simulink model "s_hover_lqr"  (Simulink 7.7)
settings: Solver=ode4  StartTime=0.0  StopTime=20  FixedStep=0.001  RelTol=1e-3
undefined symbols (not defined in the file or in its folder): CMD_RATE_LIMIT, K, K_AMP, KMIO, V_bias, VMAX_AMP, VMAX_DAC
libraries: simulink_extras x7
settings Model: Creator=hpineros  LastModifiedBy=alumno4  ExtModeTrigDuration=10000  TunableVars=A,B,C,CMD_RATE_LIMIT,D,INT_JOYSTICK_SAT_LOWER,INT_JOYSTICK_SAT_UPPER,JOYSTICK_X_DZ,JOYSTICK_Y_DZ,Jp,Jr,Jy,K,K_AMP,K_EC_P,K_EC_R,K_EC_Y,K_JOYSTICK_X,K_JOYSTICK_Y,Kf,Ktc,Ktn,Q,R,VMAX_AMP,VMAX_DAC,V_bias,g,l,wcf,zetaf  TunableVarsStorageClass=Auto,Auto,Auto,Auto,Auto,Auto,Auto,Auto,Auto,Auto,Auto,Auto,Auto,Auto,Auto,Auto,Auto,Auto,Auto,Auto,Auto,Auto,Auto,Auto,Auto,Auto,Auto,Auto,Auto,Auto,Auto  TunableVarsTypeQualifier=,,,,,,,,,,,,,,,,,,,,,,,,,,,,,,
settings SolverCC: PositivePriorityOrder=on
settings OptimizationCC: InlineParams=on  InitFltsAndDblsToZero=on
settings DebuggingCC: SaveWithParameterizedLinksMsg=none  StrictBusMsg=Warning
settings RTWCC: SystemTargetFile=quarc_windows.tlc  TemplateMakefile=quarc_default_tmf  Description=QuaRC Win32 Target  ProcessScript=quarc_windows_make_rtw_hook
settings STFCustomTargetCC: TargetFcnLib=ansi_tfl_tmw.mat  TargetPreCompLibLocation=C:\PROGRA~2\QUARC\lib\2011a\windows\release  FunctionExecutionProfile=off  GeneratePreprocessorConditionals=Disable all  SystemTargetFile=quarc_windows.tlc
settings GRTTargetCC: TargetFcnLib=ansi_tfl_tmw.mat  TargetPreCompLibLocation=C:\PROGRA~2\QUARC\lib\2011a\windows\release  ParMdlRefBuildCompliant=off  CompOptLevelCompliant=off  MatFileLogging=off  ExtMode=on  ExtModeMexFile=quarc_comm

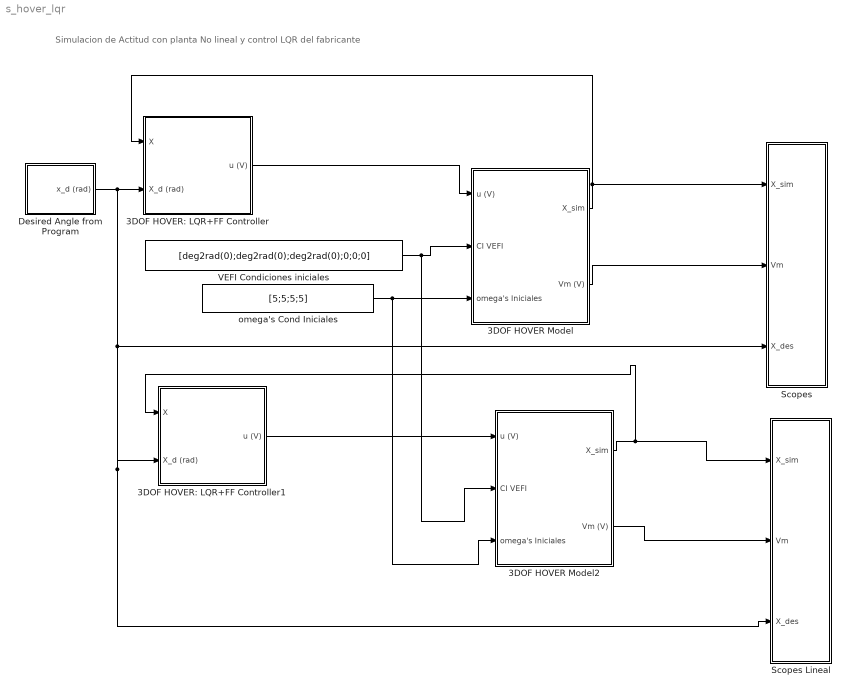
== system s_hover_lqr ==
  note: Simulacion de Actitud con planta No lineal y control LQR del fabricante
  3DOF HOVER Model : Subsystem
  3DOF HOVER Model2 : Subsystem
  3DOF HOVER: LQR+FF Controller : Subsystem
  3DOF HOVER: LQR+FF Controller1 : Subsystem
  Desired Angle from Program : Subsystem
  Scopes : Subsystem
  Scopes Lineal : Subsystem
  VEFI Condiciones iniciales : Constant  Value=[deg2rad(0);deg2rad(0);deg2rad(0);0;0;0]
  omega's Cond Iniciales : Constant  Value=[5;5;5;5]
  wires:
  Desired Angle from Program/1(x_d (rad)) -> 3DOF HOVER: LQR+FF Controller/2(X_d (rad)), Scopes/3(X_des), 3DOF HOVER: LQR+FF Controller1/2(X_d (rad)), Scopes Lineal/3(X_des)
  3DOF HOVER Model/2(Vm (V)) -> Scopes/2(Vm)
  3DOF HOVER: LQR+FF Controller/1(u (V)) -> 3DOF HOVER Model/1(u (V))
  3DOF HOVER Model/1(X_sim) -> Scopes/1(X_sim), 3DOF HOVER: LQR+FF Controller/1(X)
  VEFI Condiciones iniciales/1 -> 3DOF HOVER Model/2(CI VEFI), 3DOF HOVER Model2/2(CI VEFI)
  omega's Cond Iniciales/1 -> 3DOF HOVER Model/3(omega's Iniciales), 3DOF HOVER Model2/3(omega's Iniciales)
  3DOF HOVER Model2/1(X_sim) -> Scopes Lineal/1(X_sim), 3DOF HOVER: LQR+FF Controller1/1(X)
  3DOF HOVER Model2/2(Vm (V)) -> Scopes Lineal/2(Vm)
  3DOF HOVER: LQR+FF Controller1/1(u (V)) -> 3DOF HOVER Model2/1(u (V))

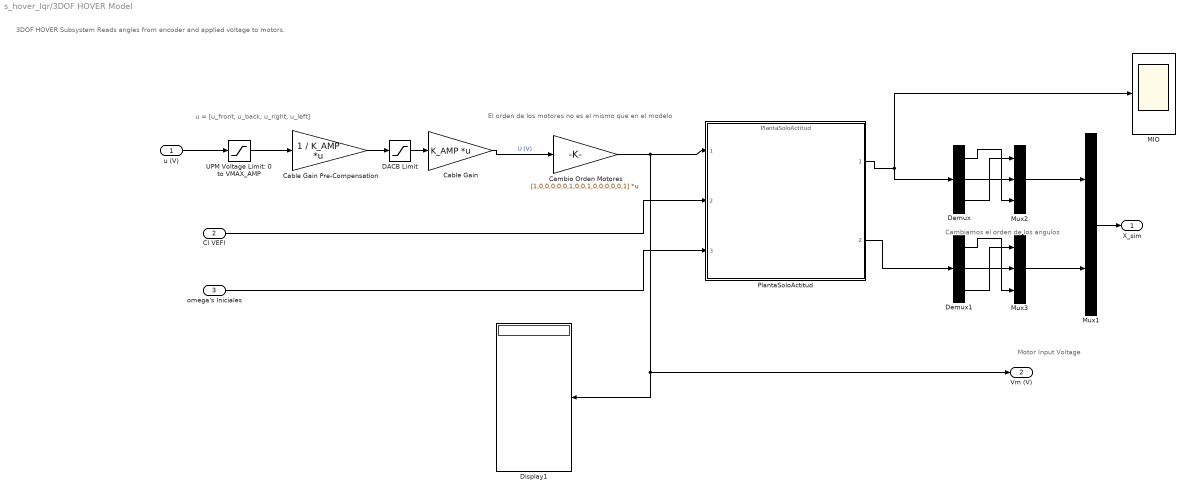
== system s_hover_lqr/3DOF HOVER Model ==
  note: Cambiamos el orden de los angulos
  note: 3DOF HOVER Subsystem
      | Reads angles from encoder and applied voltage to motors.
  note: Motor Input Voltage
  note: u = [u_front, u_back, u_right, u_left]
  note: El orden de los motores no es el mismo que en el modelo
  u (V) : Inport
  CI VEFI : Inport  Port=2
  omega's Iniciales : Inport  Port=3
  Cable Gain : Gain  Gain=K_AMP  Multiplication=Matrix(K*u)  SaturateOnIntegerOverflow=on  OutDataTypeStr=Inherit: Same as input  ParamDataTypeStr=Inherit: Same as input
  Cable Gain Pre-Compensation : Gain  Gain=1 / K_AMP  Multiplication=Matrix(K*u)  SaturateOnIntegerOverflow=on  OutDataTypeStr=Inherit: Same as input  ParamDataTypeStr=Inherit: Same as input
  Cambio Orden Motores : Gain  Gain=[1,0,0,0;0,0,1,0;0,1,0,0;0,0,0,1]  Multiplication=Matrix(K*u)  SaturateOnIntegerOverflow=on  OutDataTypeStr=Inherit: Same as input  ParamDataTypeStr=Inherit: Same as input
  DACB Limit : Saturate  UpperLimit=VMAX_DAC  LowerLimit=-VMAX_DAC
  Demux : Demux  Outputs=3
  Demux1 : Demux  Outputs=3
  Display1 : Display
  "MIO " : Scope
      settings: TickLabels=on  TimeRange=20  YMin=0.00325  YMax=0.0075  DataFormat=Array
  Mux1 : Mux  Inputs=2
  Mux2 : Mux  Inputs=3
  Mux3 : Mux  Inputs=3
  PlantaSoloActitud : ModelReference  ModelNameDialog=PlantaSoloActitud  SimulationMode=Normal  ModelReferenceVersion=1.26  CopyOfModelName=PlantaSoloActitud  DefaultDataLogging=on
  UPM Voltage Limit: 0 to VMAX_AMP : Saturate  UpperLimit=VMAX_AMP  LowerLimit=0
  X_sim : Outport
  Vm (V) : Outport  Port=2
  wires:
  Mux1/1 -> X_sim/1
  Cable Gain/1 -> Cambio Orden Motores/1  "U (V)"
  DACB Limit/1 -> Cable Gain/1
  u (V)/1 -> UPM Voltage Limit: 0 to VMAX_AMP/1
  UPM Voltage Limit: 0 to VMAX_AMP/1 -> Cable Gain Pre-Compensation/1
  Cable Gain Pre-Compensation/1 -> DACB Limit/1
  CI VEFI/1 -> PlantaSoloActitud/2
  omega's Iniciales/1 -> PlantaSoloActitud/3
  PlantaSoloActitud/1 -> "MIO "/1, Demux/1
  PlantaSoloActitud/2 -> Demux1/1
  Demux/2 -> Mux2/2
  Demux/3 -> Mux2/1
  Demux/1 -> Mux2/3
  Demux1/2 -> Mux3/2
  Demux1/3 -> Mux3/1
  Demux1/1 -> Mux3/3
  Mux3/1 -> Mux1/2
  Mux2/1 -> Mux1/1
  Cambio Orden Motores/1 -> PlantaSoloActitud/1, Vm (V)/1, Display1/1

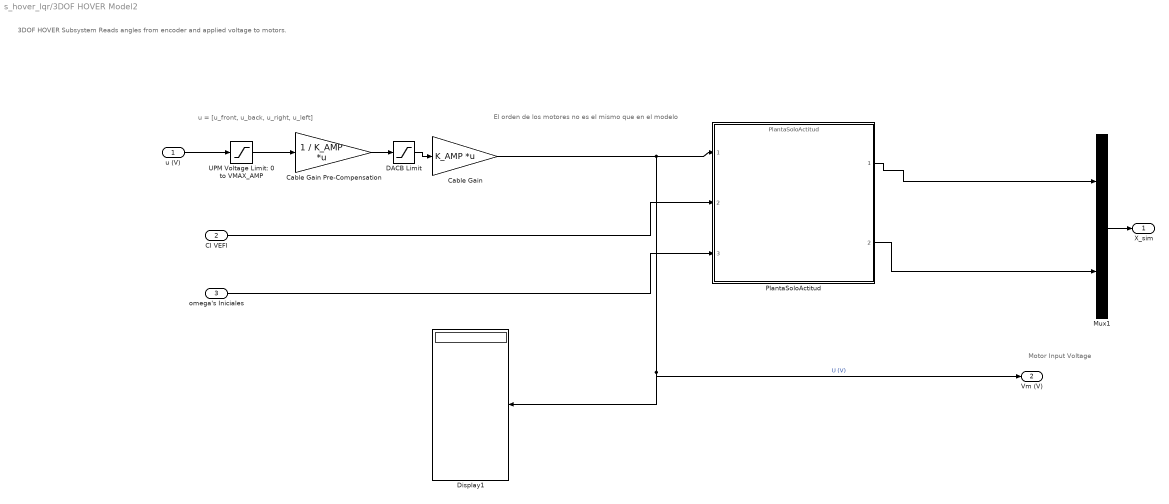
== system s_hover_lqr/3DOF HOVER Model2 ==
  note: 3DOF HOVER Subsystem
      | Reads angles from encoder and applied voltage to motors.
  note: Motor Input Voltage
  note: u = [u_front, u_back, u_right, u_left]
  note: El orden de los motores no es el mismo que en el modelo
  u (V) : Inport
  CI VEFI : Inport  Port=2
  omega's Iniciales : Inport  Port=3
  Cable Gain : Gain  Gain=K_AMP  Multiplication=Matrix(K*u)  SaturateOnIntegerOverflow=on  OutDataTypeStr=Inherit: Same as input  ParamDataTypeStr=Inherit: Same as input
  Cable Gain Pre-Compensation : Gain  Gain=1 / K_AMP  Multiplication=Matrix(K*u)  SaturateOnIntegerOverflow=on  OutDataTypeStr=Inherit: Same as input  ParamDataTypeStr=Inherit: Same as input
  DACB Limit : Saturate  UpperLimit=VMAX_DAC  LowerLimit=-VMAX_DAC
  Display1 : Display
  Mux1 : Mux  Inputs=2
  PlantaSoloActitud : ModelReference  ModelNameDialog=PlantaSoloActitud  SimulationMode=Normal  ModelReferenceVersion=1.26  CopyOfModelName=PlantaSoloActitud  DefaultDataLogging=off
  UPM Voltage Limit: 0 to VMAX_AMP : Saturate  UpperLimit=VMAX_AMP  LowerLimit=0
  X_sim : Outport
  Vm (V) : Outport  Port=2
  wires:
  Mux1/1 -> X_sim/1
  Cable Gain/1 -> PlantaSoloActitud/1, Vm (V)/1, Display1/1  "U (V)"
  DACB Limit/1 -> Cable Gain/1
  u (V)/1 -> UPM Voltage Limit: 0 to VMAX_AMP/1
  UPM Voltage Limit: 0 to VMAX_AMP/1 -> Cable Gain Pre-Compensation/1
  Cable Gain Pre-Compensation/1 -> DACB Limit/1
  CI VEFI/1 -> PlantaSoloActitud/2
  omega's Iniciales/1 -> PlantaSoloActitud/3
  PlantaSoloActitud/1 -> Mux1/1
  PlantaSoloActitud/2 -> Mux1/2

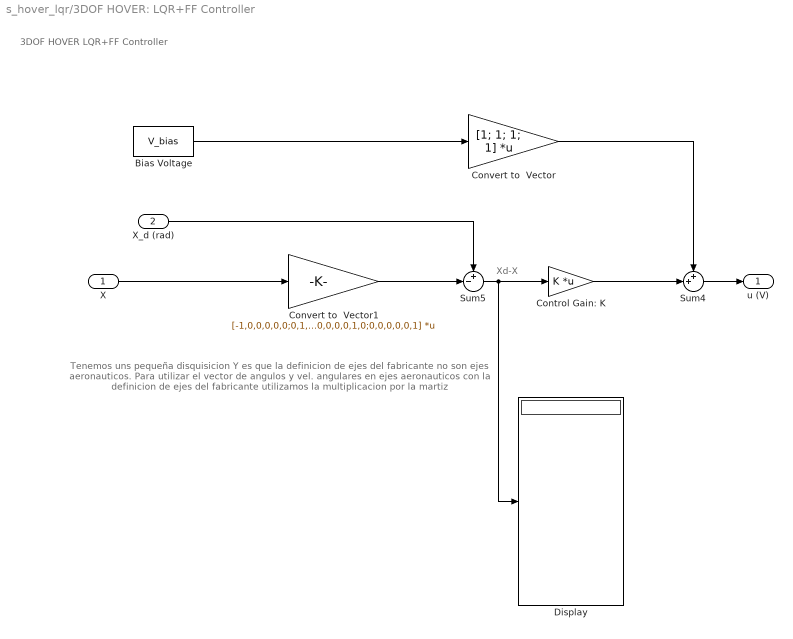
== system s_hover_lqr/3DOF HOVER: LQR+FF Controller ==
  note: Xd-X
  note: 3DOF HOVER LQR+FF Controller
  note: Tenemos uns pequeña disquisicion
      | Y es que la definicion de ejes del fabricante no son ejes aeronauticos.
      | Para utilizar el vector de angulos y vel. angulares en ejes aeronauticos
      | con la definicion de ejes del fabricante utilizamos la multiplicacion por la martiz
  X : Inport
  X_d (rad) : Inport  Port=2
  Bias Voltage : Constant  Value=V_bias
  Control Gain: K : Gain  Gain=K  Multiplication=Matrix(K*u)
  Convert to  Vector : Gain  Gain=[1; 1; 1; 1]  Multiplication=Matrix(K*u)
  Convert to  Vector1 : Gain  Gain=[-1,0,0,0,0,0;0,1,0,0,0,0;0,0,1,0,0,0;0,0,0,-1,0,0;0,0,0,0,1,0;0,0,0,0,0,1]  Multiplication=Matrix(K*u)
  Display : Display
  Sum4 : Sum  Inputs=++|
  Sum5 : Sum  Inputs=+-|
  u (V) : Outport
  wires:
  Sum5/1 -> Control Gain: K/1, Display/1
  X_d (rad)/1 -> Sum5/1
  Convert to  Vector/1 -> Sum4/1
  Control Gain: K/1 -> Sum4/2
  Bias Voltage/1 -> Convert to  Vector/1
  Sum4/1 -> u (V)/1
  Convert to  Vector1/1 -> Sum5/2
  X/1 -> Convert to  Vector1/1

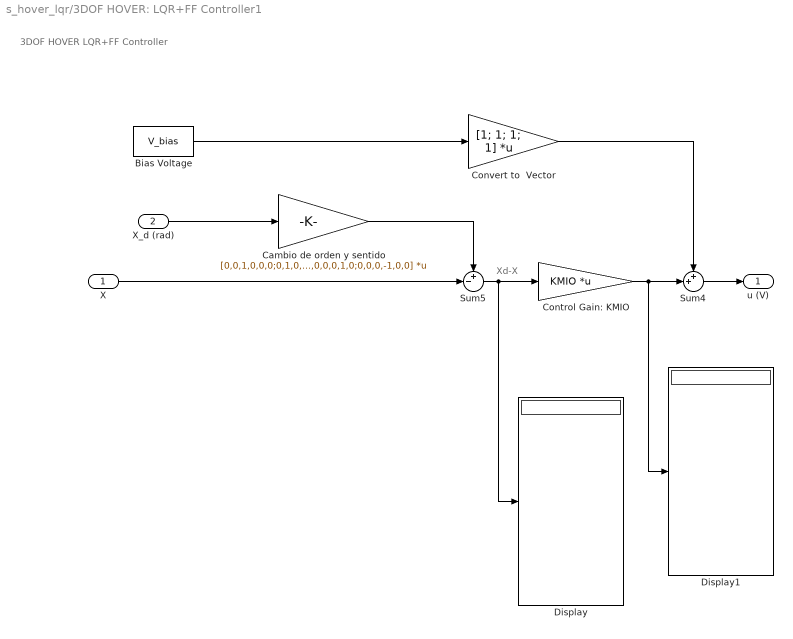
== system s_hover_lqr/3DOF HOVER: LQR+FF Controller1 ==
  note: Xd-X
  note: 3DOF HOVER LQR+FF Controller
  X : Inport
  X_d (rad) : Inport  Port=2
  Bias Voltage : Constant  Value=V_bias
  Cambio de orden y sentido : Gain  Gain=[0,0,1,0,0,0;0,1,0,0,0,0;-1,0,0,0,0,0;0,0,0,0,0,1;0,0,0,0,1,0;0,0,0,-1,0,0]  Multiplication=Matrix(K*u)
  Control Gain: KMIO : Gain  Gain=KMIO  Multiplication=Matrix(K*u) (u vector)
  Convert to  Vector : Gain  Gain=[1; 1; 1; 1]  Multiplication=Matrix(K*u)
  Display : Display
  Display1 : Display
  Sum4 : Sum  Inputs=++|
  Sum5 : Sum  Inputs=+-|
  u (V) : Outport
  wires:
  Sum5/1 -> Control Gain: KMIO/1, Display/1
  X_d (rad)/1 -> Cambio de orden y sentido/1
  Convert to  Vector/1 -> Sum4/1
  Control Gain: KMIO/1 -> Sum4/2, Display1/1
  Bias Voltage/1 -> Convert to  Vector/1
  Sum4/1 -> u (V)/1
  X/1 -> Sum5/2
  Cambio de orden y sentido/1 -> Sum5/1

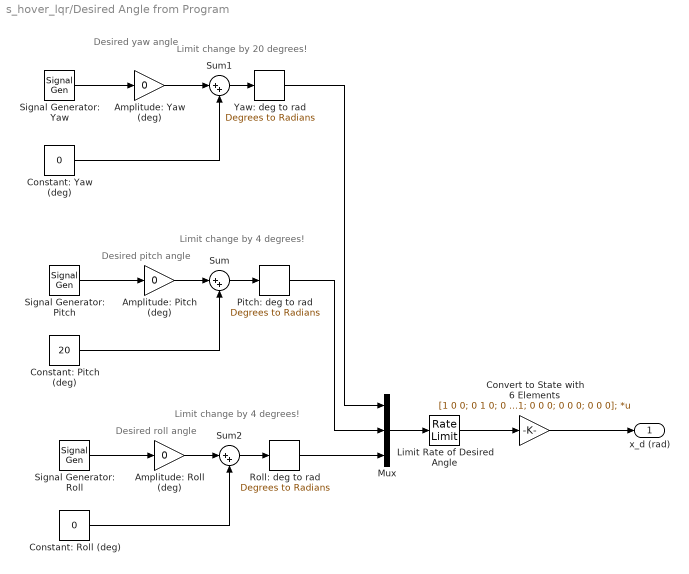
== system s_hover_lqr/Desired Angle from Program ==
  note: Limit change by
      | 4 degrees!
  note: Limit change by
      | 20 degrees!
  note: Limit change by
      | 4 degrees!
  note: Desired roll angle
  note: Desired pitch angle
  note: Desired yaw angle
  Amplitude: Pitch (deg) : Gain  Gain=0
  Amplitude: Roll (deg) : Gain  Gain=0
  Amplitude: Yaw (deg) : Gain  Gain=0
  Constant: Pitch (deg) : Constant  Value=20
  Constant: Roll (deg) : Constant  Value=0
  Constant: Yaw (deg) : Constant  Value=0
  Convert to State with 6 Elements : Gain  Gain=[1 0 0; 0 1 0; 0 0 1; 0 0 0; 0 0 0; 0 0 0];  Multiplication=Matrix(K*u)
  Limit Rate of Desired Angle : RateLimiter  RisingSlewLimit=CMD_RATE_LIMIT  FallingSlewLimit=-CMD_RATE_LIMIT
  Mux : Mux  Inputs=3
  Pitch: deg to rad : simulink_extras/Transformations/Degrees to Radians  SystemSampleTime=-1
  Roll: deg to rad : simulink_extras/Transformations/Degrees to Radians  SystemSampleTime=-1
  Signal Generator: Pitch : SignalGenerator  WaveForm=square  Frequency=0.0000001
  Signal Generator: Roll : SignalGenerator  WaveForm=square  Frequency=0.08
  Signal Generator: Yaw : SignalGenerator  WaveForm=square  Frequency=0.04
  Sum : Sum  Inputs=|++
  Sum1 : Sum  Inputs=|++
  Sum2 : Sum  Inputs=|++
  Yaw: deg to rad : simulink_extras/Transformations/Degrees to Radians  SystemSampleTime=-1
  x_d (rad) : Outport
  wires:
  Convert to State with 6 Elements/1 -> x_d (rad)/1
  Limit Rate of Desired Angle/1 -> Convert to State with 6 Elements/1
  Roll: deg to rad/1 -> Mux/3
  Pitch: deg to rad/1 -> Mux/2
  Yaw: deg to rad/1 -> Mux/1
  Sum2/1 -> Roll: deg to rad/1
  Signal Generator: Roll/1 -> Amplitude: Roll (deg)/1
  Amplitude: Roll (deg)/1 -> Sum2/1
  Constant: Roll (deg)/1 -> Sum2/2
  Sum/1 -> Pitch: deg to rad/1
  Signal Generator: Pitch/1 -> Amplitude: Pitch (deg)/1
  Amplitude: Pitch (deg)/1 -> Sum/1
  Constant: Pitch (deg)/1 -> Sum/2
  Sum1/1 -> Yaw: deg to rad/1
  Signal Generator: Yaw/1 -> Amplitude: Yaw (deg)/1
  Amplitude: Yaw (deg)/1 -> Sum1/1
  Constant: Yaw (deg)/1 -> Sum1/2
  Mux/1 -> Limit Rate of Desired Angle/1

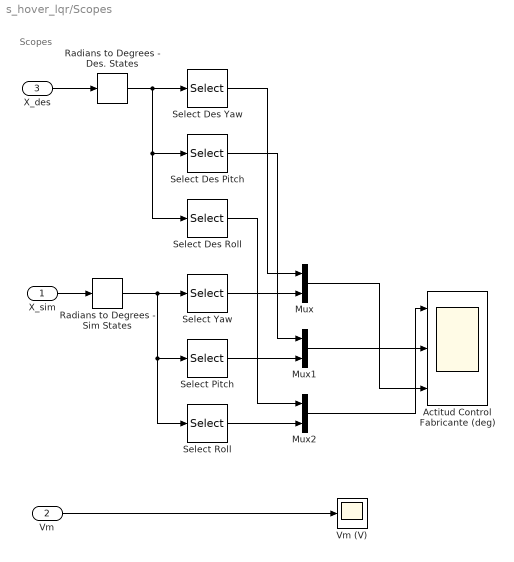
== system s_hover_lqr/Scopes ==
  note: Scopes
  X_sim : Inport
  Vm : Inport  Port=2
  X_des : Inport  Port=3
  Actitud Control Fabricante (deg) : Scope  NumInputPorts=3
      settings: TickLabels=on  TimeRange=20  YMin=0~0~0  YMax=1.4e-008~20~0.0008  SaveName=Ensayo1
  Mux : Mux  Inputs=2
  Mux1 : Mux  Inputs=2
  Mux2 : Mux  Inputs=2
  Radians to Degrees - Des. States : simulink_extras/Transformations/Radians to Degrees  SystemSampleTime=-1
  Radians to Degrees - Sim States : simulink_extras/Transformations/Radians to Degrees  SystemSampleTime=-1
  Select Des Pitch : Selector  InputPortWidth=6  IndexOptions=Index vector (dialog)  Indices=2  OutputSizes=1
  Select Des Roll : Selector  InputPortWidth=6  IndexOptions=Index vector (dialog)  Indices=3  OutputSizes=1
  Select Des Yaw : Selector  InputPortWidth=6  IndexOptions=Index vector (dialog)  Indices=1  OutputSizes=1
  Select Pitch : Selector  InputPortWidth=6  IndexOptions=Index vector (dialog)  Indices=2  OutputSizes=1
  Select Roll : Selector  InputPortWidth=6  IndexOptions=Index vector (dialog)  Indices=3  OutputSizes=1
  Select Yaw : Selector  InputPortWidth=6  IndexOptions=Index vector (dialog)  Indices=1  OutputSizes=1
  Vm (V) : Scope
      settings: TickLabels=on  TimeRange=20  YMin=0  YMax=25  SaveName=ScopeData4  DataFormat=Array
  wires:
  Select Des Roll/1 -> Mux2/1
  Select Des Pitch/1 -> Mux1/1
  Select Des Yaw/1 -> Mux/1
  Radians to Degrees - Des. States/1 -> Select Des Roll/1, Select Des Pitch/1, Select Des Yaw/1
  Select Roll/1 -> Mux2/2
  Select Pitch/1 -> Mux1/2
  Select Yaw/1 -> Mux/2
  Radians to Degrees - Sim States/1 -> Select Roll/1, Select Pitch/1, Select Yaw/1
  Vm/1 -> Vm (V)/1
  X_sim/1 -> Radians to Degrees - Sim States/1
  X_des/1 -> Radians to Degrees - Des. States/1
  Mux/1 -> Actitud Control Fabricante (deg)/3
  Mux2/1 -> Actitud Control Fabricante (deg)/1
  Mux1/1 -> Actitud Control Fabricante (deg)/2

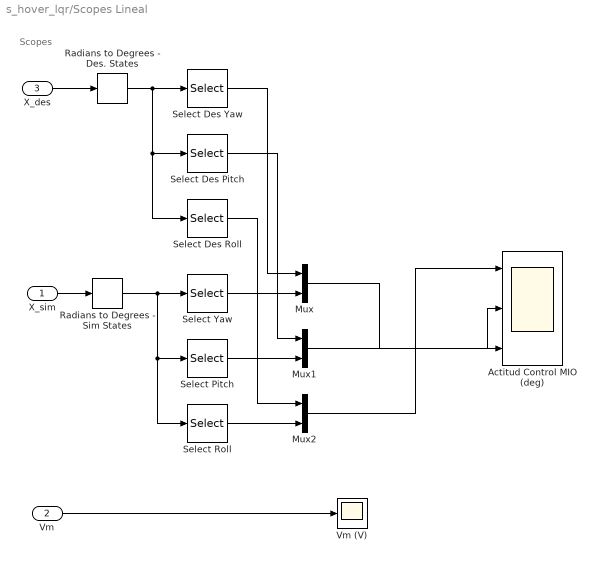
== system s_hover_lqr/Scopes Lineal ==
  note: Scopes
  X_sim : Inport
  Vm : Inport  Port=2
  X_des : Inport  Port=3
  Actitud Control MIO (deg) : Scope  NumInputPorts=3
      settings: TickLabels=on  TimeRange=20  YMin=0~-0~-0.00175  YMax=0.00055~20~0  SaveName=Ensayo1
  Mux : Mux  Inputs=2
  Mux1 : Mux  Inputs=2
  Mux2 : Mux  Inputs=2
  Radians to Degrees - Des. States : simulink_extras/Transformations/Radians to Degrees  SystemSampleTime=-1
  Radians to Degrees - Sim States : simulink_extras/Transformations/Radians to Degrees  SystemSampleTime=-1
  Select Des Pitch : Selector  InputPortWidth=6  IndexOptions=Index vector (dialog)  Indices=2  OutputSizes=1
  Select Des Roll : Selector  InputPortWidth=6  IndexOptions=Index vector (dialog)  Indices=3  OutputSizes=1
  Select Des Yaw : Selector  InputPortWidth=6  IndexOptions=Index vector (dialog)  Indices=1  OutputSizes=1
  Select Pitch : Selector  InputPortWidth=6  IndexOptions=Index vector (dialog)  Indices=2  OutputSizes=1
  Select Roll : Selector  InputPortWidth=6  IndexOptions=Index vector (dialog)  Indices=3  OutputSizes=1
  Select Yaw : Selector  InputPortWidth=6  IndexOptions=Index vector (dialog)  Indices=1  OutputSizes=1
  Vm (V) : Scope
      settings: TickLabels=on  TimeRange=20  YMin=0  YMax=25  SaveName=ScopeData4  DataFormat=Array
  wires:
  Select Des Roll/1 -> Mux2/1
  Select Des Pitch/1 -> Mux1/1
  Select Des Yaw/1 -> Mux/1
  Radians to Degrees - Des. States/1 -> Select Des Roll/1, Select Des Pitch/1, Select Des Yaw/1
  Select Roll/1 -> Mux2/2
  Select Pitch/1 -> Mux1/2
  Select Yaw/1 -> Mux/2
  Radians to Degrees - Sim States/1 -> Select Roll/1, Select Pitch/1, Select Yaw/1
  Vm/1 -> Vm (V)/1
  X_sim/1 -> Radians to Degrees - Sim States/1
  X_des/1 -> Radians to Degrees - Des. States/1
  Mux/1 -> Actitud Control MIO (deg)/3
  Mux2/1 -> Actitud Control MIO (deg)/1
  Mux1/1 -> Actitud Control MIO (deg)/2
